simulink model "PSI7"  (R2016b)
settings: Solver=FixedStepAuto  StartTime=0.0  StopTime=inf  FixedStep=0.1  RelTol=1e-3
libraries: instrumentlib x2, aerolibanimutils x1
settings Model: Creator=Oleksandr  LastModifiedBy=Oleksandr

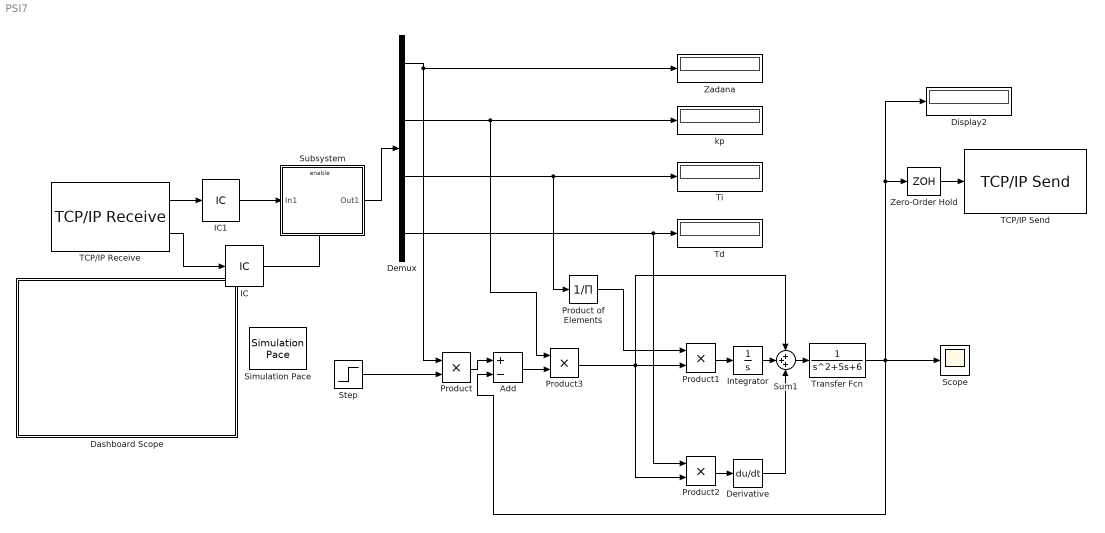
== system PSI7 ==
  Add : Sum  Inputs=+-
  Dashboard Scope : Subsystem  DialogController=hmiCreateDDGDialog  IsWebBlock=on  mask(MWDashboardBlock){webBlockId=4283cdf4-46ca-4549-8ffa-01565ead0560, webBlockType=sdiscope, ShowInitialText=on, HMISrcModelName=PSI7}
      mask prompts: webBlockId "WebBlock Id"; webBlockType "WebBlock Type"; HMISrcModelName "Source Model"
      mask help: SimulinkHMI:dialogs:HMIScopeDialogDesc
      mask Help: helpview([docroot '/mapfiles/simulink.map'], 'hmi_scope')
      mask Display:
      | if strcmp(get_param(bdroot(gcb),'BlockDiagramType'), 'library')
      |     image([(matlabroot) '/toolbox/simulink/hmi/icons/DashboardScope.png']);
      | end
  Demux : Demux
  Derivative : Derivative
  Display2 : Display
  IC : InitialCondition
  IC1 : InitialCondition  Value=[0 1 1 0]
  Integrator : Integrator
  Product{,1..3} (4 alike) : Product
  Product of Elements : Product  Inputs=/
  Scope : Scope
  Simulation Pace : aerolibanimutils/Simulation Pace  SimulationPace=1  SleepMode=MATLAB Thread  OutputPaceError=off  SampleTime=0.1
  Step : Step  SampleTime=0
  Subsystem : Subsystem
  Sum1 : Sum  Inputs=+++
  TCP/IP Receive : instrumentlib/TCP//IP Receive  Host=192.168.0.155  Port=2137  DataSize=4  EnableBlockingMode=off  Timeout=10  SampleTime=0.1  DataType=double  ByteOrder=BigEndian
  TCP/IP Send : instrumentlib/TCP//IP Send  Host=192.168.0.155  Port=2137  EnableBlockingMode=on  Timeout=10  ByteOrder=BigEndian
  Td : Display
  Ti : Display
  Transfer Fcn : TransferFcn  Denominator=[1 5 6]
  Zadana : Display
  Zero-Order Hold : ZeroOrderHold  SampleTime=0.1
  kp : Display
  wires:
  Transfer Fcn/1 -> Display2/1, Zero-Order Hold/1, Scope/1, Add/2
  Step/1 -> Product/2
  Subsystem/1(Out1) -> Demux/1
  Demux/1 -> Product/1, Zadana/1
  Product1/1 -> Integrator/1
  Product/1 -> Add/1
  TCP/IP Receive/2 -> IC/1
  IC/1 -> Subsystem/Enable
  Product of Elements/1 -> Product1/1
  TCP/IP Receive/1 -> IC1/1
  IC1/1 -> Subsystem/1(In1)
  Zero-Order Hold/1 -> TCP/IP Send/1
  Demux/2 -> Product3/1, kp/1
  Demux/3 -> Product of Elements/1, Ti/1
  Demux/4 -> Product2/1, Td/1
  Product2/1 -> Derivative/1
  Sum1/1 -> Transfer Fcn/1
  Derivative/1 -> Sum1/3
  Integrator/1 -> Sum1/2
  Add/1 -> Product3/2
  Product3/1 -> Sum1/1, Product2/2, Product1/2

== system PSI7/Dashboard Scope ==

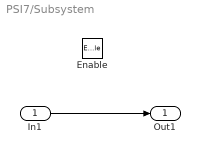
== system PSI7/Subsystem ==
  In1 : Inport
  Enable : EnablePort
  Out1 : Outport
  wires:
  In1/1 -> Out1/1
